simulink model "tank"  (R2022b)
settings: Solver=VariableStepAuto  StartTime=0.0  StopTime=80  RelTol=1e-3
values from neighbouring files (symbols this model uses):
  x0 = [0;0;0]    [tank_params.m]
settings Model: Creator=super  LastModifiedBy=15043
settings SolverCC: AlgebraicLoopSolver=TrustRegion
settings DataIOCC: ReturnWorkspaceOutputs=off
settings DebuggingCC: UnconnectedInputMsg=warning  UnconnectedOutputMsg=warning  UnconnectedLineMsg=warning  SFMachineParentedDataDiag=warning  ArithmeticOperatorsInVariantConditions=warning
settings ModelReferenceCC: EnableRefExpFcnMdlSchedulingChecks=on
settings SFSimCC: SimUseLocalCustomCode=off  CustomCodeUndefinedFunction=UseInterfaceOnly
settings RTWCC: RTWUseLocalCustomCode=off

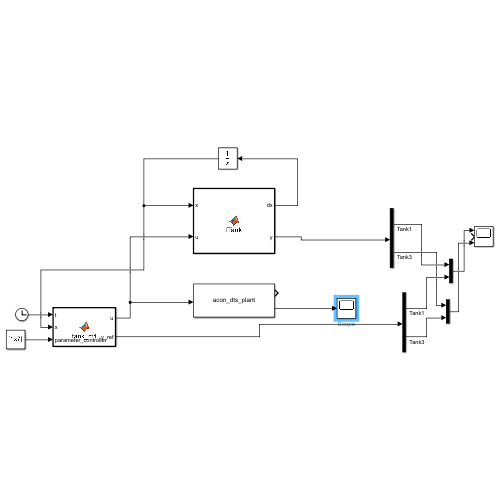
[thumbnail: Simulink's stored preview of the top-level diagram]
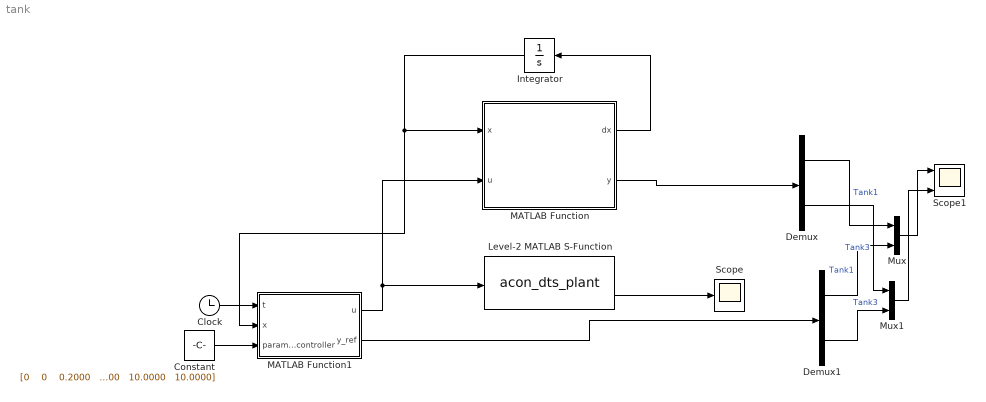
== system tank ==
  Clock : Clock
  Constant : Constant  Value="[0    0    0.2000    0.2500   80.0000   10.0000   10.0000]"
  Demux : Demux  Outputs=2
  Demux1 : Demux  Outputs=2
  Integrator : Integrator  InitialCondition=x0  ZeroCross=off
  Level-2 MATLAB S-Function : M-S-Function  FunctionName=acon_dts_plant  Parameters=x0
  MATLAB Function : MATLAB Function  TreatAsAtomicUnit=on
  MATLAB Function1 : MATLAB Function  TreatAsAtomicUnit=on
  Mux : Mux  Inputs=2
  Mux1 : Mux  Inputs=2
  Scope : Scope
  Scope1 : Scope  NumInputPorts=3
  wires:
  MATLAB Function/1(dx) -> Integrator/1
  Integrator/1 -> MATLAB Function/1(x), MATLAB Function1/2(x)
  Level-2 MATLAB S-Function/2 -> Scope/1
  MATLAB Function/2(y) -> Demux/1
  MATLAB Function1/1(u) -> Level-2 MATLAB S-Function/1, MATLAB Function/2(u)
  Clock/1 -> MATLAB Function1/1(t)
  Demux/1 -> Mux/1  "Tank1"
  MATLAB Function1/2(y_ref) -> Demux1/1
  Demux1/1 -> Mux/2  "Tank1"
  Demux/2 -> Mux1/1  "Tank3"
  Demux1/2 -> Mux1/2  "Tank3"
  Mux/1 -> Scope1/1
  Mux1/1 -> Scope1/3
  Constant/1 -> MATLAB Function1/3(parameter_controller)

== matlab function tank/MATLAB Function1 ==
  data: u output; t input; x input; y_ref output; parameter_controller input
function [u,y_ref]  = tank_ctrl(t,x, parameter_controller)
   
    x1 = x(1,:);
    x2 = x(2,:);
    x3 = x(3,:);
    
   y10 = parameter_controller(1);
   y20 = parameter_controller(2);
   y1T = parameter_controller(3);
   y2T = parameter_controller(4);
   T = parameter_controller(5);
   p1 = parameter_controller(6);
   p2 = parameter_controller(7);


   u1 = (4377800396407898125*T^3*((5520653160719109*x1)/562949953421312)^(1/2) + 8522395762053812846592*t^2*y10 - 8522395762053812846592*t^2*y1T + 2840798587351270948864*p1*t^3*y10 - 2840798587351270948864*p1*t^3*y1T - 8522395762053812846592*T*t*y10 + 8522395762053812846592*T*t*y1T + 7155462338586337500*T^3*abs(x1 - x2)^(1/2)*sign(x1 - x2) - 1420399293675635474432*T^3*p1*x1 + 1420399293675635474432*T^3*p1*y10 - 4261197881026906423296*T*p1*t^2*y10 + 4261197881026906423296*T*p1*t^2*y1T)/(92233720368547758080000*T^3);
   u2 = (2160707084972626875*T^3*((5520653160719109*x3)/562949953421312)^(1/2) + 4261197881026906423296*t^2*y20 - 4261197881026906423296*t^2*y2T + 1420399293675635474432*p2*t^3*y20 - 1420399293675635474432*p2*t^3*y2T - 4261197881026906423296*T*t*y20 + 4261197881026906423296*T*t*y2T - 3577731169293168750*T^3*abs(x2 - x3)^(1/2)*sign(x2 - x3) - 710199646837817737216*T^3*p2*x3 + 710199646837817737216*T^3*p2*y20 - 2130598940513453211648*T*p2*t^2*y20 + 2130598940513453211648*T*p2*t^2*y2T)/(46116860184273879040000*T^3);

   u = [u1; u2];
   y1_ref = (3*t^2/T^2 - 2*t^3/T^3)*(y1T - y10)+ y10;
   y2_ref = (3*t^2/T^2 - 2*t^3/T^3)*(y2T - y20)+ y20;
   y_ref = [y1_ref; y2_ref;];
end

== matlab function tank/MATLAB Function ==
  data: x input; dx output; u input; y output; par parameter
function [dx, y] = fTank( x, u, par )
    
    % The water levels of the tanks x1,x2 and x3 represent the state 
    % variables of the system.
    x1 = x(1);
    x2 = x(2);
    x3 = x(3);

    % symbolic parameter values
    % At is the cross sectional area of the tanks
    % Av is the cross sectional area of the valves
    % a12, a23, a10, a30I are the correction factors due to internal friction
    %               of the fluid, pipe friction, deformation of water jet
    % g is the gravity
    At      = par(1);
    Av      = par(2);
    a12     = par(3);
    a23     = par(4);
    a10     = par(5);
    a30I    = par(6);
    g       = par(7);
    
%     % Input vector
%     Qp1 = u(1);     % Pump flow of tank 1
%     Qp2 = u(2);     % Pump flow of tank 3    

    % Initialize the xdot vector
    fx = zeros(3,1);

    fx(1) = -(2^(1/2)*Av*a10*(g*x1)^(1/2) + 2^(1/2)*Av*a12*g^(1/2)*sign(x1 - x2)*abs(x1 - x2)^(1/2))/At;
    fx(2) = (2^(1/2)*Av*a12*g^(1/2)*sign(x1 - x2)*abs(x1 - x2)^(1/2) - 2^(1/2)*Av*a23*g^(1/2)*sign(x2 - x3)*abs(x2 - x3)^(1/2))/At;
    fx(3) = - (2^(1/2)*Av*a30I*(g*x3)^(1/2) - 2^(1/2)*Av*a23*g^(1/2)*sign(x2 - x3)*abs(x2 - x3)^(1/2))/At;
    
    g1 = [1/At; 0; 0;];
    g2 = [0; 0; 1/At ];
    gx = [g1 g2];
        
    dx = fx + gx*u;
    
%     dx(1) =  -(2^(1/2)*Av*a10*(g*x1)^(1/2) - Qp1 + 2^(1/2)*Av*a12*g^(1/2)*sign(x1 - x2)*abs(x1 - x2)^(1/2))/At;
%     dx(2) = (2^(1/2)*Av*a12*g^(1/2)*sign(x1 - x2)*abs(x1 - x2)^(1/2) - 2^(1/2)*Av*a23*g^(1/2)*sign(x2 - x3)*abs(x2 - x3)^(1/2))/At;
%     dx(3) = (Qp2 - 2^(1/2)*Av*a30I*(g*x3)^(1/2) + 2^(1/2)*Av*a23*g^(1/2)*sign(x2 - x3)*abs(x2 - x3)^(1/2))/At;

    y = [x1; x3];
end
